simulink model "T2_LDI"  (R2022a)
settings: Solver=VariableStepAuto  StartTime=0.0  StopTime=20  RelTol=1e-3
values from neighbouring files (symbols this model uses):
  A = state_space.A    [T2_LDI_PreLoadFcn.m]
  B = state_space.B    [T2_LDI_PreLoadFcn.m]
  C = state_space.C    [T2_LDI_PreLoadFcn.m]
  C11 = -0.1    [T2_PreLoadFcn.m]
  C21 = -0.1    [T2_PreLoadFcn.m]
  D = state_space.D    [T2_LDI_PreLoadFcn.m]
undefined symbols (not defined in the file or in its folder): I_C, I_D, sysID_DAQ
libraries: slpidlib x2
settings Model: Creator=user  LastModifiedBy=user
settings DataIOCC: ReturnWorkspaceOutputs=off

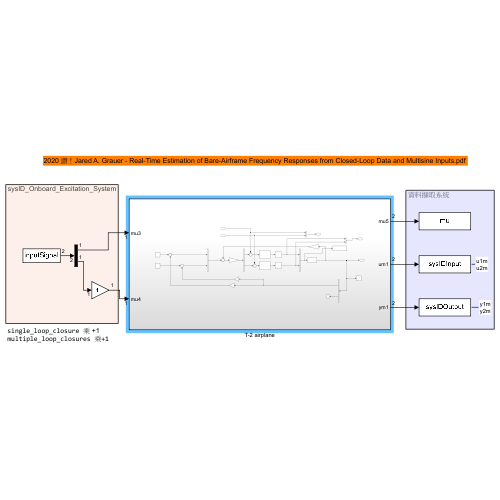
[thumbnail: Simulink's stored preview of the top-level diagram]
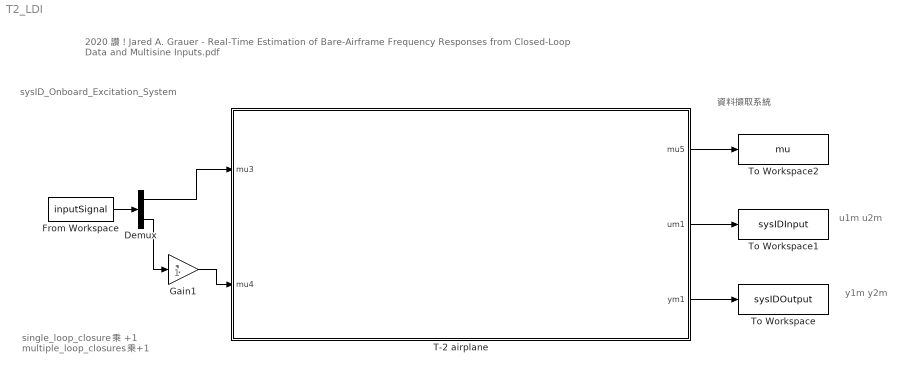
== system T2_LDI ==
  note: 資料擷取系統
  note: 1
  note: 2020 讚！Jared A. Grauer - Real-Time Estimation of Bare-Airframe Frequency Responses from Closed-Loop Data and Multisine Inputs.pdf
  note: single_loop_closure 乘 +1
      | multiple_loop_closures 乘+1
  note: y1m
      | y2m
  note: sysID_Onboard_Excitation_System
  note: u1m
      | u2m
  Demux : Demux  Outputs=2
  From Workspace : FromWorkspace  VariableName=inputSignal  OutputAfterFinalValue=Holding final value
  Gain1 : Gain
  T-2 airplane : Subsystem
  To Workspace : ToWorkspace  VariableName=sysIDOutput  SaveFormat=Timeseries  SampleTime=sysID_DAQ.sampleTime
  To Workspace1 : ToWorkspace  VariableName=sysIDInput  SaveFormat=Timeseries  SampleTime=sysID_DAQ.sampleTime
  To Workspace2 : ToWorkspace  VariableName=mu  SaveFormat=Timeseries  SampleTime=sysID_DAQ.sampleTime
  wires:
  T-2 airplane/2(um1) -> To Workspace1/1
  Demux/1 -> T-2 airplane/1(mu3)
  T-2 airplane/1(mu5) -> To Workspace2/1
  Demux/2 -> Gain1/1
  From Workspace/1 -> Demux/1
  Gain1/1 -> T-2 airplane/2(mu4)
  T-2 airplane/3(ym1) -> To Workspace/1

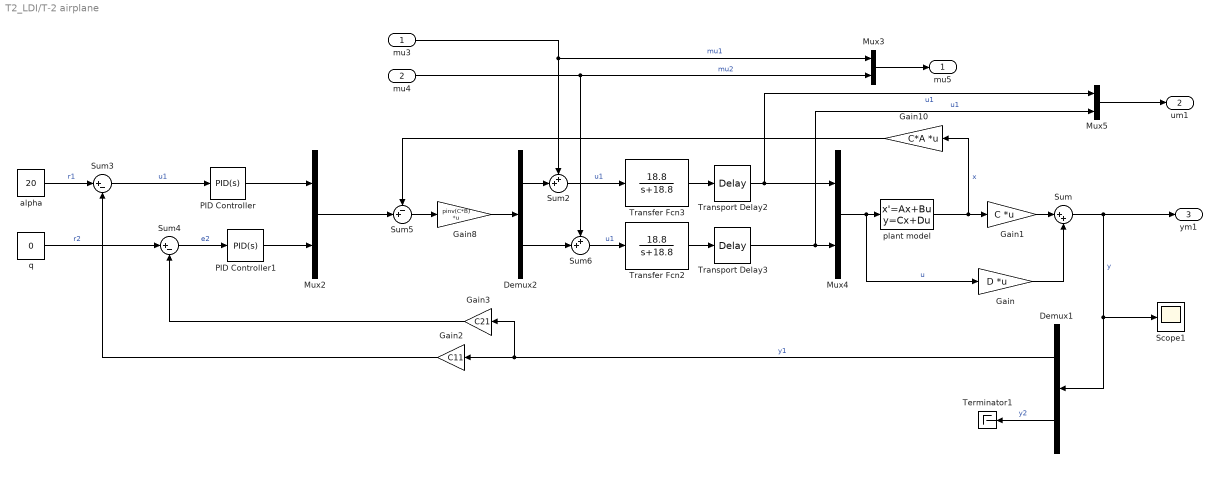
== system T2_LDI/T-2 airplane ==
  mu3 : Inport
  mu4 : Inport  Port=2
  Demux1 : Demux  Outputs=2
  Demux2 : Demux  Outputs=2
  Gain : Gain  Gain=D  Multiplication=Matrix(K*u) (u vector)
  Gain1 : Gain  Gain=C  Multiplication=Matrix(K*u) (u vector)
  Gain10 : Gain  Gain=C*A  Multiplication=Matrix(K*u) (u vector)
  Gain2 : Gain  Gain=C11
  Gain3 : Gain  Gain=C21
  Gain8 : Gain  Gain=pinv(C*B)  Multiplication=Matrix(K*u) (u vector)
  Mux{2..5} (4 alike) : Mux  Inputs=2
  PID Controller : slpidlib/PID Controller  Controller=PID  Form=Parallel  TimeDomain=Continuous-time  UseExternalTs=off  SampleTime=-1  IntegratorMethod=Forward Euler  FilterMethod=Forward Euler  ControllerParametersSource=internal  P=53.7615961684536  I=271.568663354112  UseKiTs=off  D=2.56387260378157  N=5306.2109363596  UseFilter=on  TunerSelectOption=Transfer Function Based (PID Tuner App)  InitialConditionSource=internal  InitialConditionForIntegrator=0  InitialConditionForFilter=0  DifferentiatorICPrevScaledInput=0  ExternalReset=none  TrackingMode=off  Kt=1  LimitOutput=off  SatLimitsSource=internal  UpperSaturationLimit=inf  LowerSaturationLimit=-inf  LinearizeAsGain=on  AntiWindupMode=none  Kb=1  POutMin=[]  POutMax=[]  IOutMin=[]  IOutMax=[]  DOutMin=[]  DOutMax=[]  NOutMin=[]  NOutMax=[]  SumOutMin=[]  SumOutMax=[]  SaturationOutMin=[]  SaturationOutMax=[]  PParamMin=[]  PParamMax=[]  IParamMin=[]  IParamMax=[]  DParamMin=[]  DParamMax=[]  NParamMin=[]  NParamMax=[]  KbParamMin=[]  KbParamMax=[]  KtParamMin=[]  KtParamMax=[]  KbOutMin=[]  KbOutMax=[]  KtOutMin=[]  KtOutMax=[]  IntegratorOutMin=[]  IntegratorOutMax=[]  FilterOutMin=[]  FilterOutMax=[]  SumI1OutMin=[]  SumI1OutMax=[]  SumI2OutMin=[]  SumI2OutMax=[]  SumI3OutMin=[]  SumI3OutMax=[]  SumI4OutMin=[]  SumI4OutMax=[]  SumDOutMin=[]  SumDOutMax=[]  DifferentiatorOutMin=[]  DifferentiatorOutMax=[]  FilterDiffOutCoefMin=[]  FilterDiffOutCoefMax=[]  ReciprocalOutMin=[]  ReciprocalOutMax=[]  SumDenOutMin=[]  SumDenOutMax=[]  SumNumOutMin=[]  SumNumOutMax=[]  DivideOutMin=[]  DivideOutMax=[]  UdiffTsProdOutMin=[]  UdiffTsProdOutMax=[]  NTsProdOutMin=[]  NTsProdOutMax=[]  UintegralTsProdOutMin=[]  UintegralTsProdOutMax=[]  UngainTsProdOutMin=[]  UngainTsProdOutMax=[]  IntegratorContinuousStateAttributes=''  IntegratorStateMustResolveToSignalObject=off  IntegratorRTWStateStorageClass=Auto  FilterContinuousStateAttributes=''  FilterStateMustResolveToSignalObject=off  FilterRTWStateStorageClass=Auto  ParallelPVariant=InternalParameters  IdealPVariant=Disabled  IVariant=InternalParameters  DVariant=InternalParameters  IntegratorVariant=Continuous  SatVariant=Disabled  AWVariant=Passthrough  PCopyVariant=Disabled  TRVariant=Disabled  FdbkBlocksVariant=Forward  IdealPFdbkVariant=Disabled  SatFdbkVariant=Disabled  DerivativeFilterVariant=ContFilter  NVariant=InternalParameters  NCopyVariant=Disabled  FilterICVariant=InternalICsFilter  IntegratorICVariant=InternalICs  ExternalResetVariant=Disabled  TRSumVariant=Passthrough  SumFdbkVariant=Disabled  SumVariant=Sum_PID  TsampFilterVariant=InternalTs  TsampNgainVariant=Passthrough  TsampIntegralVariant=Passthrough  ExternalSaturationOutDataTypeStr=Inherit: Same as second input  aMode=0
  PID Controller1 : slpidlib/PID Controller  Controller=PID  Form=Parallel  TimeDomain=Continuous-time  UseExternalTs=off  SampleTime=-1  IntegratorMethod=Forward Euler  FilterMethod=Forward Euler  ControllerParametersSource=internal  P=53.7615961684536  I=271.568663354112  UseKiTs=off  D=2.56387260378157  N=5306.2109363596  UseFilter=on  TunerSelectOption=Transfer Function Based (PID Tuner App)  InitialConditionSource=internal  InitialConditionForIntegrator=0  InitialConditionForFilter=0  DifferentiatorICPrevScaledInput=0  ExternalReset=none  TrackingMode=off  Kt=1  LimitOutput=off  SatLimitsSource=internal  UpperSaturationLimit=inf  LowerSaturationLimit=-inf  LinearizeAsGain=on  AntiWindupMode=none  Kb=1  POutMin=[]  POutMax=[]  IOutMin=[]  IOutMax=[]  DOutMin=[]  DOutMax=[]  NOutMin=[]  NOutMax=[]  SumOutMin=[]  SumOutMax=[]  SaturationOutMin=[]  SaturationOutMax=[]  PParamMin=[]  PParamMax=[]  IParamMin=[]  IParamMax=[]  DParamMin=[]  DParamMax=[]  NParamMin=[]  NParamMax=[]  KbParamMin=[]  KbParamMax=[]  KtParamMin=[]  KtParamMax=[]  KbOutMin=[]  KbOutMax=[]  KtOutMin=[]  KtOutMax=[]  IntegratorOutMin=[]  IntegratorOutMax=[]  FilterOutMin=[]  FilterOutMax=[]  SumI1OutMin=[]  SumI1OutMax=[]  SumI2OutMin=[]  SumI2OutMax=[]  SumI3OutMin=[]  SumI3OutMax=[]  SumI4OutMin=[]  SumI4OutMax=[]  SumDOutMin=[]  SumDOutMax=[]  DifferentiatorOutMin=[]  DifferentiatorOutMax=[]  FilterDiffOutCoefMin=[]  FilterDiffOutCoefMax=[]  ReciprocalOutMin=[]  ReciprocalOutMax=[]  SumDenOutMin=[]  SumDenOutMax=[]  SumNumOutMin=[]  SumNumOutMax=[]  DivideOutMin=[]  DivideOutMax=[]  UdiffTsProdOutMin=[]  UdiffTsProdOutMax=[]  NTsProdOutMin=[]  NTsProdOutMax=[]  UintegralTsProdOutMin=[]  UintegralTsProdOutMax=[]  UngainTsProdOutMin=[]  UngainTsProdOutMax=[]  IntegratorContinuousStateAttributes=''  IntegratorStateMustResolveToSignalObject=off  IntegratorRTWStateStorageClass=Auto  FilterContinuousStateAttributes=''  FilterStateMustResolveToSignalObject=off  FilterRTWStateStorageClass=Auto  ParallelPVariant=InternalParameters  IdealPVariant=Disabled  IVariant=InternalParameters  DVariant=InternalParameters  IntegratorVariant=Continuous  SatVariant=Disabled  AWVariant=Passthrough  PCopyVariant=Disabled  TRVariant=Disabled  FdbkBlocksVariant=Forward  IdealPFdbkVariant=Disabled  SatFdbkVariant=Disabled  DerivativeFilterVariant=ContFilter  NVariant=InternalParameters  NCopyVariant=Disabled  FilterICVariant=InternalICsFilter  IntegratorICVariant=InternalICs  ExternalResetVariant=Disabled  TRSumVariant=Passthrough  SumFdbkVariant=Disabled  SumVariant=Sum_PID  TsampFilterVariant=InternalTs  TsampNgainVariant=Passthrough  TsampIntegralVariant=Passthrough  ExternalSaturationOutDataTypeStr=Inherit: Same as second input  aMode=0
  Scope1 : Scope
  Sum : Sum  Inputs=|++
  Sum2 : Sum  Inputs=++|
  Sum3 : Sum  Inputs=|+-
  Sum4 : Sum  Inputs=|+-
  Sum5 : Sum  Inputs=-+|
  Sum6 : Sum  Inputs=++|
  Terminator1 : Terminator
  Transfer Fcn2 : TransferFcn  Numerator=[18.8]  Denominator=[1 18.8]
  Transfer Fcn3 : TransferFcn  Numerator=[18.8]  Denominator=[1 18.8]
  Transport Delay2 : TransportDelay  DelayTime=0.01  InitialOutput=-1.5  BufferSize=2048
  Transport Delay3 : TransportDelay  DelayTime=0.01  InitialOutput=-1.5  BufferSize=2048
  alpha : Constant  Value=20
  plant model : StateSpace  A=A  B=B  C=I_C  D=I_D  InitialCondition=0
  q : Constant  Value=0
  mu5 : Outport
  um1 : Outport  Port=2
  ym1 : Outport  Port=3
  wires:
  Gain2/1 -> Sum3/2
  Demux2/2 -> Sum6/2
  alpha/1 -> Sum3/1  "r1"
  Gain8/1 -> Demux2/1
  mu4/1 -> Mux3/2, Sum6/1  "mu2"
  Demux2/1 -> Sum2/2
  plant model/1 -> Gain10/1, Gain1/1  "x"
  q/1 -> Sum4/1  "r2"
  Sum3/1 -> PID Controller/1  "u1"
  Mux4/1 -> Gain/1, plant model/1  "u"
  Mux5/1 -> um1/1
  Mux3/1 -> mu5/1
  Gain10/1 -> Sum5/1
  Sum5/1 -> Gain8/1
  Sum4/1 -> PID Controller1/1  "e2"
  mu3/1 -> Sum2/1, Mux3/1  "mu1"
  Demux1/1 -> Gain3/1, Gain2/1  "y1"
  Mux2/1 -> Sum5/2
  Sum6/1 -> Transfer Fcn2/1  "u1"
  Sum2/1 -> Transfer Fcn3/1  "u1"
  Gain3/1 -> Sum4/2
  Sum/1 -> Scope1/1, Demux1/1, ym1/1  "y"
  Gain/1 -> Sum/2
  Gain1/1 -> Sum/1
  PID Controller/1 -> Mux2/1
  PID Controller1/1 -> Mux2/2
  Transfer Fcn2/1 -> Transport Delay3/1
  Transfer Fcn3/1 -> Transport Delay2/1
  Transport Delay2/1 -> Mux5/1, Mux4/1  "u1"
  Transport Delay3/1 -> Mux5/2, Mux4/2  "u1"
  Demux1/2 -> Terminator1/1  "y2"
